simulink model "INDUCTIONMACHINE"  (R2024b)
settings: Solver=VariableStepAuto  StartTime=0.0  StopTime=0.5  RelTol=1e-3
libraries: spsRMSLib x2, spsAsynchronousMachineSIUnitsLib x1, spsPower3phInstantaneousLib x1, spsThreePhaseVIMeasurementLib x1, spsThreePhaseSourceLib x1, spsVoltageMeasurementLib x1, sps_lib x1
settings Model: Creator=495ka  LastModifiedBy=495ka

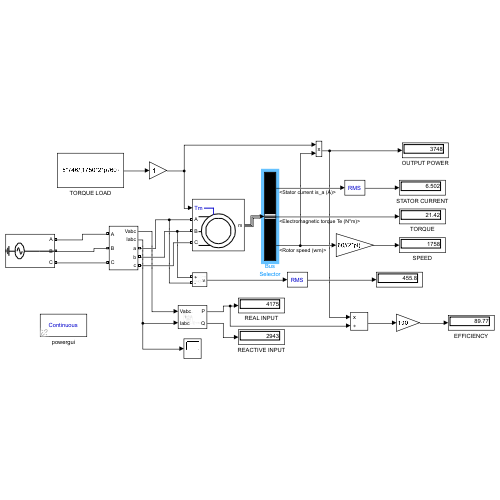
[thumbnail: Simulink's stored preview of the top-level diagram]
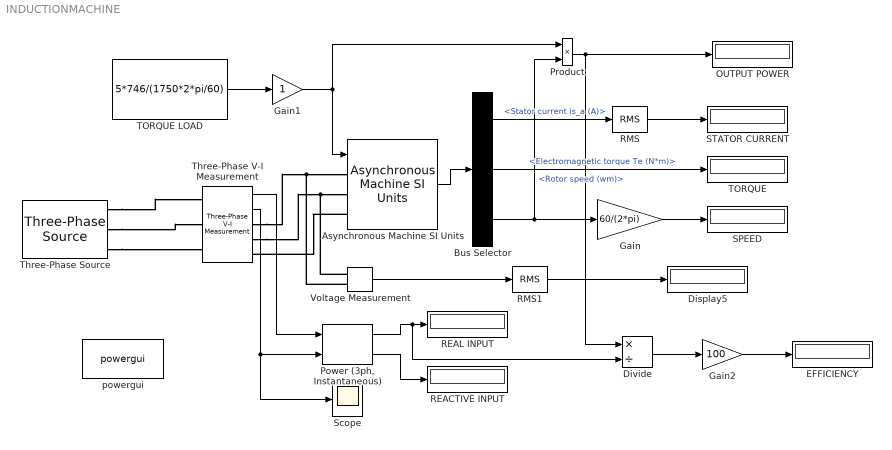
== system INDUCTIONMACHINE ==
  Asynchronous Machine SI Units : spsAsynchronousMachineSIUnitsLib/Asynchronous Machine SI Units  RotorType=Squirrel-cage  PresetModel="01:  5 HP   460 V 60Hz 1750 RPM"  MechanicalLoad=Torque Tm  ShowDetailedParameters=on  ReferenceFrame=Rotor  Units=SI  MeasurementBus=off  NominalParameters=[3730 460 60]  VoltageRatio=1  Stator=[1.115 0.005974]  Rotor=[1.083 0.005974]  Cage1=[0.4155 0.002066]  Cage2=[0.4168 0.0003495]  Lm=0.2037  Mechanical=[0.02 0.005752 2]  PolePairs=2  InitialConditions=[1 0 0 0 0 0 0 0]  SimulateSaturation=off  Saturation=[14.03593122, 27.81365428, 53.79336849, 72.68890987, 97.98006896, 148.6815601, 215.7428561, 302.9841135, 428.7778367 ; 230, 322, 414, 460, 506, 552, 598, 644, 690]  LoadFlowParameters=1492000  TsPowergui=0  TsBlock=-1  IterativeModel=Trapezoidal non iterative  IterativeDiscreteModel=Trapezoidal non iterative  Pmec=1.492e+006
  Bus Selector : BusSelector  OutputSignals=Stator measurements.Stator current is_a (A),Mechanical.Electromagnetic torque Te (N*m),Mechanical.Rotor speed (wm)
  Display5 : Display
  Divide : Product  Inputs=*/
  EFFICIENCY : Display
  Gain : Gain  Gain=60/(2*pi)
  Gain1 : Gain
  Gain2 : Gain  Gain=100
  OUTPUT POWER : Display
  "Power (3ph, Instantaneous)" : spsPower3phInstantaneousLib/Power (3ph, Instantaneous)
  Product : Product
  REACTIVE INPUT : Display
  REAL INPUT : Display
  RMS : spsRMSLib/RMS  TrueRMS=on  Freq=60  RMSInit=120  Ts=0
  RMS1 : spsRMSLib/RMS  TrueRMS=on  Freq=60  RMSInit=120  Ts=0
  SPEED : Display
  STATOR CURRENT : Display
  Scope : Scope
  TORQUE : Display
  TORQUE LOAD : Constant  Value=5*746/(1750*2*pi/60)
  Three-Phase V-I Measurement : spsThreePhaseVIMeasurementLib/Three-Phase V-I Measurement  VoltageMeasurement=phase-to-ground  SetLabelV=off  LabelV=Vabc  Vpu=off  VpuLL=off  CurrentMeasurement=yes  SetLabelI=off  LabelI=Iabc  Ipu=off  Pbase=100e6  Vbase=500e3  OutputType=Complex  PhasorSimulation=off  PSBequivalent=0
  Three-Phase Source : spsThreePhaseSourceLib/Three-Phase Source  InternalConnection=Yg  VoltagePhases=off  Voltage=460  PhaseAngle=0  Voltage_phases=[25e3 25e3 25e3]/sqrt(3)  PhaseAngles_phases=[0 -120 +120]  Frequency=60  NonIdealSource=off  SpecifyImpedance=off  Resistance=0.8929  Inductance=16.58e-3  ShortCircuitLevel=100e6  BaseVoltage=25e3  XRratio=7  BusType=swing  Pref=10e3  Qref=0  Prefabc=[10e3, 10e3, 10e3]  Qrefabc=[0, 0, 0]  Qmin=-inf  Qmax=inf
  Voltage Measurement : spsVoltageMeasurementLib/Voltage Measurement  PhasorSimulation=off  OutputType=Complex  PSBequivalent=0
  powergui : sps_lib/powergui  Priority=1  SimulationMode=Continuous  SampleTime=50e-6  frequency=60  Iterations=50  frequencyindice=60  Pbase=100e6  ErrMax=1e-4  UnitsV=kV  UnitsW=MW  buscounter=0  FunctionMessages=off  echomessages=off  EnableUseOfTLC=off  CurrentSourceSwitches=off  DisableSnubberDevices=off  DisableRonSwitches=off  DisableVfSwitches=off  DisplayEquations=off  AutomaticDiscreteSolvers=off  SolverType=Tustin/Backward Euler (TBE)  Interpol=off  ExternalGateDelay=off  methode=off  Ts=100  x0status=blocks  SPID=on  SwTol=0  HookPort=off  NonlinearTolerance=1e-4  nMaxIteration=100  ContinueOnMaxIteration=off  RestoreLinks=warning  ResistiveCurrentMeasurement=off  Frange=[0:2:500]  Ylog=off  Xlog=on  ShowGrid=off  save=off  variable=ZData  structure=0  ZoomFFT=off  StartTime=0.0  cycles=1  DisplayStyle=1  fundamental=60  FreqAxis=off  MaxFrequency=1000  frequencyindicesteady=1  RmsSteady=1  display=off
  wires:
  TORQUE LOAD/1 -> Gain1/1
  Asynchronous Machine SI Units/1 -> Bus Selector/1
  Bus Selector/1 -> RMS/1  "<Stator current is_a (A)>"
  RMS/1 -> STATOR CURRENT/1
  Gain/1 -> SPEED/1
  Bus Selector/3 -> Product/2, Gain/1  "<Rotor speed (wm)>"
  Bus Selector/2 -> TORQUE/1  "<Electromagnetic torque Te (N*m)>"
  Gain1/1 -> Asynchronous Machine SI Units/1, Product/1
  Product/1 -> OUTPUT POWER/1, Divide/1
  Three-Phase V-I Measurement/1 -> "Power (3ph, Instantaneous)"/1
  Three-Phase V-I Measurement/2 -> Scope/1, "Power (3ph, Instantaneous)"/2
  "Power (3ph, Instantaneous)"/1 -> Divide/2, REAL INPUT/1
  "Power (3ph, Instantaneous)"/2 -> REACTIVE INPUT/1
  Voltage Measurement/1 -> RMS1/1
  RMS1/1 -> Display5/1
  Gain2/1 -> EFFICIENCY/1
  Divide/1 -> Gain2/1
  connections:
  Three-Phase Source/RConn1 -- Three-Phase V-I Measurement/LConn1
  Three-Phase Source/RConn2 -- Three-Phase V-I Measurement/LConn2
  Three-Phase Source/RConn3 -- Three-Phase V-I Measurement/LConn3
  Three-Phase V-I Measurement/RConn1 -- Voltage Measurement/LConn2 -- Asynchronous Machine SI Units/LConn1
  Three-Phase V-I Measurement/RConn2 -- Voltage Measurement/LConn1 -- Asynchronous Machine SI Units/LConn2
  Asynchronous Machine SI Units/LConn3 -- Three-Phase V-I Measurement/RConn3
